simulink model "reference_model_prob6"  (R2020a)
settings: Solver=VariableStepAuto  StartTime=0.0  StopTime=10.0  RelTol=1e-3
settings Model: Creator=sonal  LastModifiedBy=sonal
settings DataIOCC: SaveOutput=off  SaveTime=off

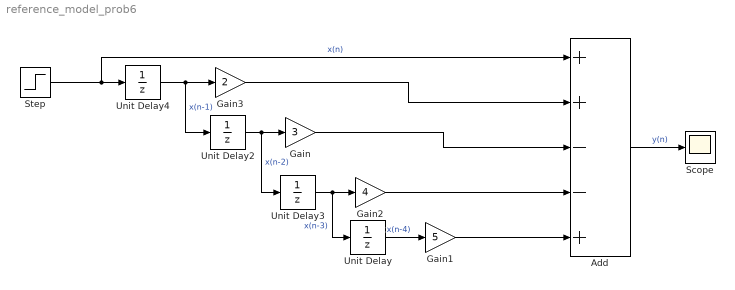
== system reference_model_prob6 ==
  Add : Sum  Inputs=++--+
  Gain : Gain  Gain=3
  Gain1 : Gain  Gain=5
  Gain2 : Gain  Gain=4
  Gain3 : Gain  Gain=2
  Scope : Scope
  Step : Step  SampleTime=0
  Unit Delay{,2..4} (4 alike) : UnitDelay  SampleTime=-1  HasFrameUpgradeWarning=on
  wires:
  Gain3/1 -> Add/2
  Step/1 -> Unit Delay4/1, Add/1  "x(n)"
  Gain2/1 -> Add/4
  Unit Delay/1 -> Gain1/1  "x(n-4)"
  Unit Delay3/1 -> Gain2/1, Unit Delay/1  "x(n-3)"
  Unit Delay2/1 -> Gain/1, Unit Delay3/1  "x(n-2)"
  Gain/1 -> Add/3
  Gain1/1 -> Add/5
  Unit Delay4/1 -> Gain3/1, Unit Delay2/1  "x(n-1)"
  Add/1 -> Scope/1  "y(n)"
